simulink model "RW_control"  (R2021b)
settings: Solver=ode45  StartTime=0.0  StopTime=33600  RelTol=1e-3  EnableMultiTasking=on
libraries: sim_operations x6
settings Model: Creator=Sanny  LastModifiedBy=ajbar
settings SolverCC: AlgebraicLoopSolver=TrustRegion
settings DataIOCC: ReturnWorkspaceOutputs=off
settings OptimizationCC: LifeSpan=inf
settings DebuggingCC: SFUnexpectedBacktrackingDiag=warning  SFNoUnconditionalDefaultTransitionDiag=warning  SFMachineParentedDataDiag=warning  ArithmeticOperatorsInVariantConditions=warning
settings SFSimCC: SimUseLocalCustomCode=off  CustomCodeUndefinedFunction=UseInterfaceOnly
settings RTWCC: RTWUseLocalCustomCode=off
settings CodeAppCC: StateflowObjectComments=on
settings GRTTargetCC: TargetLangStandard=C89/C90 (ANSI)
settings ConfigComp: CovMetricSettings=dw  CovSaveCumulativeToWorkspaceVar=on  CovSaveSingleToWorkspaceVar=on  CovExternalEMLEnable=off

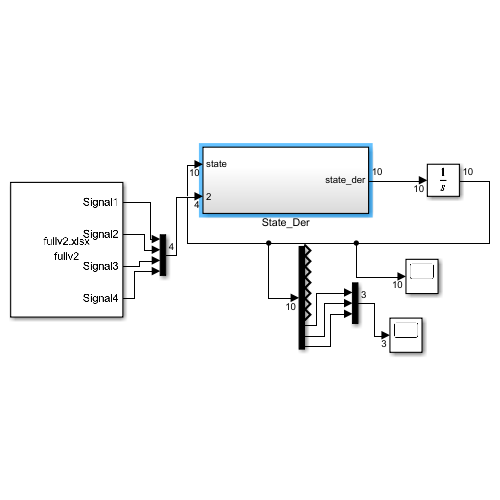
[thumbnail: Simulink's stored preview of the top-level diagram]
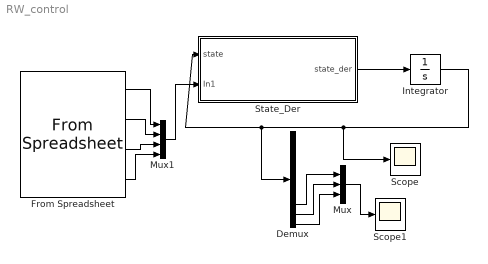
== system RW_control ==
  Demux : Demux  Outputs=10
  From Spreadsheet : FromSpreadsheet  FileName=fullv2.xlsx  SheetName=fullv2  Range=A1:E33601
  Integrator : Integrator  InitialCondition=[1 0 0 0 0 0 0 0 0 0]'
  Mux : Mux  Inputs=3
  Mux1 : Mux
  Scope : Scope
  Scope1 : Scope
  State_Der : Subsystem  Description=State consists of quat, sat_ang_vel, wheel_ang_vels
  wires:
  State_Der/1(state_der) -> Integrator/1
  Integrator/1 -> Scope/1, Demux/1, State_Der/1(state)
  Demux/8 -> Mux/1
  Demux/9 -> Mux/2
  Demux/10 -> Mux/3
  Mux/1 -> Scope1/1
  From Spreadsheet/3 -> Mux1/3
  From Spreadsheet/2 -> Mux1/2
  From Spreadsheet/4 -> Mux1/4
  From Spreadsheet/1 -> Mux1/1
  Mux1/1 -> State_Der/2(In1)

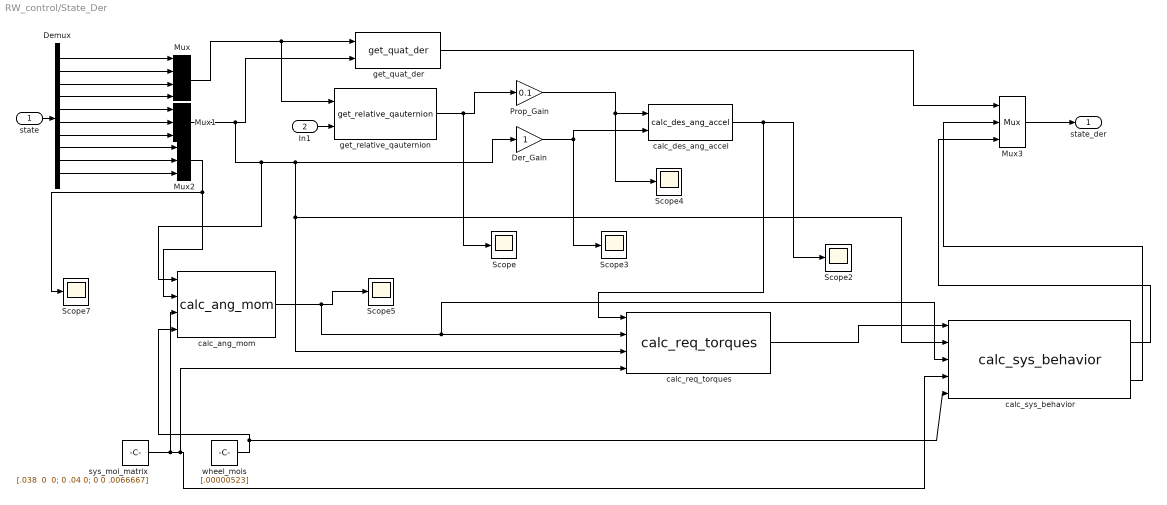
== system RW_control/State_Der ==
  state : Inport
  In1 : Inport  Port=2
  Demux : Demux  Outputs=10
  Der_Gain : Gain
  Mux : Mux
  Mux1 : Mux  Inputs=3
  Mux2 : Mux  Inputs=3
  Mux3 : Mux  Inputs=3
  Prop_Gain : Gain  Gain=0.1
  Scope{,2..5,7} (6 alike) : Scope
  calc_ang_mom : sim_operations/calc_ang_mom  SystemSampleTime=-1  VariantActivationTime=update diagram  Latency=0  AutoFrameSizeCalculation=off
  calc_des_ang_accel : sim_operations/calc_des_ang_accel  SystemSampleTime=-1  VariantActivationTime=update diagram  Latency=0  AutoFrameSizeCalculation=off
  calc_req_torques : sim_operations/calc_req_torques  SystemSampleTime=-1  VariantActivationTime=update diagram  Latency=0  AutoFrameSizeCalculation=off
  calc_sys_behavior : sim_operations/calc_sys_behavior  SystemSampleTime=-1  VariantActivationTime=update diagram  Latency=0  AutoFrameSizeCalculation=off
  get_quat_der : sim_operations/get_quat_der  SystemSampleTime=-1  VariantActivationTime=update diagram  Latency=0  AutoFrameSizeCalculation=off
  get_relative_qauternion : sim_operations/get_relative_qauternion  SystemSampleTime=-1  VariantActivationTime=update diagram  Latency=0  AutoFrameSizeCalculation=off
  sys_moi_matrix : Constant  Value="[.038  0  0; 0 .04 0; 0 0 .0066667]"
  wheel_mois : Constant  Value=[.00000523]
  state_der : Outport
  wires:
  state/1 -> Demux/1
  Demux/1 -> Mux/1
  Demux/2 -> Mux/2
  Demux/3 -> Mux/3
  Demux/4 -> Mux/4
  Demux/5 -> Mux1/1
  Demux/6 -> Mux1/2
  Demux/7 -> Mux1/3
  Demux/8 -> Mux2/1
  Demux/9 -> Mux2/2
  Demux/10 -> Mux2/3
  Mux/1 -> get_relative_qauternion/1, get_quat_der/1
  In1/1 -> get_relative_qauternion/2
  Prop_Gain/1 -> calc_des_ang_accel/1, Scope4/1
  Der_Gain/1 -> Scope3/1, calc_des_ang_accel/2
  calc_des_ang_accel/1 -> calc_req_torques/1, Scope2/1
  get_relative_qauternion/1 -> Scope/1, Prop_Gain/1
  get_quat_der/1 -> Mux3/1
  Mux3/1 -> state_der/1
  Mux1/1 -> calc_ang_mom/1, calc_sys_behavior/2, calc_req_torques/3, Der_Gain/1, get_quat_der/2
  sys_moi_matrix/1 -> calc_sys_behavior/4, calc_req_torques/4, calc_ang_mom/3
  Mux2/1 -> Scope7/1, calc_ang_mom/2
  wheel_mois/1 -> calc_sys_behavior/5, calc_ang_mom/4
  calc_ang_mom/1 -> calc_sys_behavior/3, calc_req_torques/2, Scope5/1
  calc_req_torques/1 -> calc_sys_behavior/1
  calc_sys_behavior/1 -> Mux3/3
  calc_sys_behavior/2 -> Mux3/2
